simulink model "Quad_Linear_LQR"  (R2020a)
settings: Solver=ode4  StartTime=0.0  StopTime=10.0  FixedStep=0.01  RelTol=1e-3
InitFcn:
  | QuadConstants
undefined symbols (not defined in the file or in its folder): A1, A3, B1, B3, C2, Omega
settings Model: Creator=Ali  LastModifiedBy=Ali

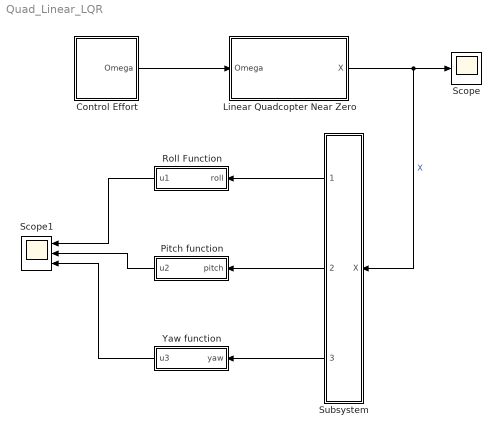
== system Quad_Linear_LQR ==
  Control Effort : Subsystem
  Linear Quadcopter Near Zero : Subsystem
  Pitch function : MATLAB Function  TreatAsAtomicUnit=on
  Roll Function : MATLAB Function  TreatAsAtomicUnit=on
  Scope : Scope
  Scope1 : Scope  NumInputPorts=3
  Subsystem : Subsystem
  Yaw function : MATLAB Function  TreatAsAtomicUnit=on
  wires:
  Control Effort/1(Omega) -> Linear Quadcopter Near Zero/1(Omega)
  Linear Quadcopter Near Zero/1(X) -> Subsystem/1(X), Scope/1  "X"
  Subsystem/1(roll) -> Roll Function/1(roll)
  Subsystem/2(pitch) -> Pitch function/1(pitch)
  Subsystem/3(yaw) -> Yaw function/1(yaw)
  Roll Function/1(u1) -> Scope1/1
  Pitch function/1(u2) -> Scope1/2
  Yaw function/1(u3) -> Scope1/3

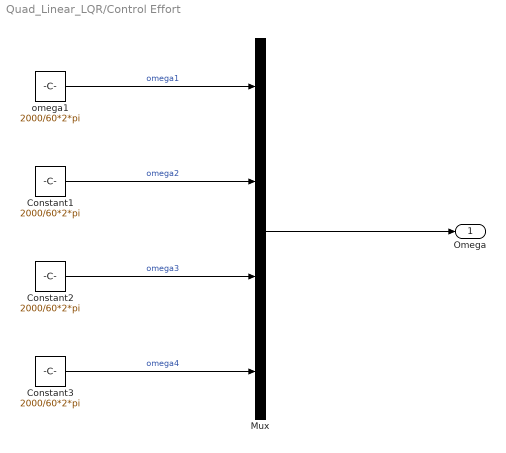
== system Quad_Linear_LQR/Control Effort ==
  Constant1 : Constant  Value=2000/60*2*pi
  Constant2 : Constant  Value=2000/60*2*pi
  Constant3 : Constant  Value=2000/60*2*pi
  Mux : Mux
  omega1 : Constant  Value=2000/60*2*pi
  Omega : Outport
  wires:
  Constant1/1 -> Mux/2  "omega2"
  Constant2/1 -> Mux/3  "omega3"
  Constant3/1 -> Mux/4  "omega4"
  omega1/1 -> Mux/1  "omega1"
  Mux/1 -> Omega/1

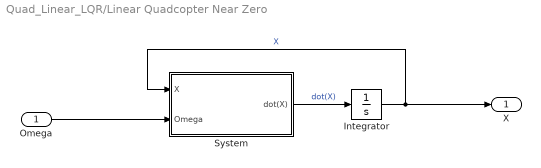
== system Quad_Linear_LQR/Linear Quadcopter Near Zero ==
  Omega : Inport
  Integrator : Integrator
  System : Subsystem
  X : Outport
  wires:
  Integrator/1 -> X/1, System/1(X)  "X"
  System/1(dot(X)) -> Integrator/1  "dot(X)"
  Omega/1 -> System/2(Omega)

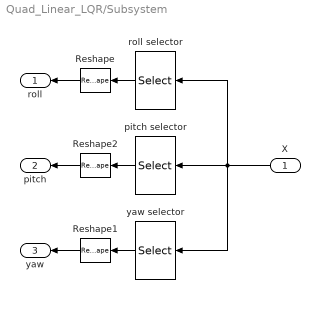
== system Quad_Linear_LQR/Subsystem ==
  X : Inport
  Reshape : Reshape  OutputDimensionality=Column vector (2-D)
  Reshape1 : Reshape  OutputDimensionality=Column vector (2-D)
  Reshape2 : Reshape  OutputDimensionality=Column vector (2-D)
  pitch selector : Selector  InputPortWidth=6  IndexOptions=Index vector (dialog)  Indices=[2 5]  OutputSizes=1
  roll selector : Selector  InputPortWidth=6  IndexOptions=Index vector (dialog)  Indices=[1 4]  OutputSizes=1
  yaw selector : Selector  InputPortWidth=6  IndexOptions=Index vector (dialog)  Indices=[3 6]  OutputSizes=1
  roll : Outport
  pitch : Outport  Port=2
  yaw : Outport  Port=3
  wires:
  X/1 -> yaw selector/1, roll selector/1, pitch selector/1
  roll selector/1 -> Reshape/1
  pitch selector/1 -> Reshape2/1
  yaw selector/1 -> Reshape1/1
  Reshape/1 -> roll/1
  Reshape2/1 -> pitch/1
  Reshape1/1 -> yaw/1

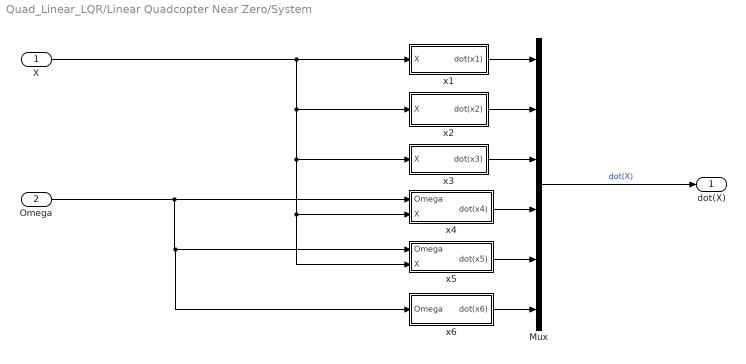
== system Quad_Linear_LQR/Linear Quadcopter Near Zero/System ==
  X : Inport
  Omega : Inport  Port=2
  Mux : Mux  Inputs=6
  x1 : Subsystem
  x2 : Subsystem
  x3 : Subsystem
  x4 : Subsystem
  x5 : Subsystem
  x6 : Subsystem
  dot(X) : Outport
  wires:
  Omega/1 -> x4/1(Omega), x6/1(Omega), x5/1(Omega)
  x6/1(dot(x6)) -> Mux/6
  x3/1(dot(x3)) -> Mux/3
  x4/1(dot(x4)) -> Mux/4
  x2/1(dot(x2)) -> Mux/2
  X/1 -> x5/2(X), x4/2(X), x3/1(X), x2/1(X), x1/1(X)
  x5/1(dot(x5)) -> Mux/5
  x1/1(dot(x1)) -> Mux/1
  Mux/1 -> dot(X)/1  "dot(X)"

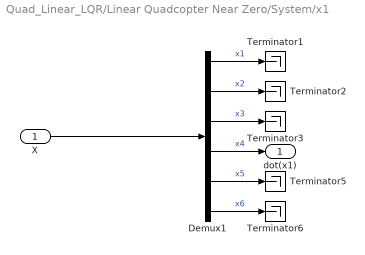
== system Quad_Linear_LQR/Linear Quadcopter Near Zero/System/x1 ==
  X : Inport
  Demux1 : Demux  Outputs=6
  Terminator{1..3,5..6} (5 alike) : Terminator
  dot(x1) : Outport
  wires:
  Demux1/4 -> dot(x1)/1  "x4"
  X/1 -> Demux1/1
  Demux1/6 -> Terminator6/1  "x6"
  Demux1/5 -> Terminator5/1  "x5"
  Demux1/3 -> Terminator3/1  "x3"
  Demux1/2 -> Terminator2/1  "x2"
  Demux1/1 -> Terminator1/1  "x1"

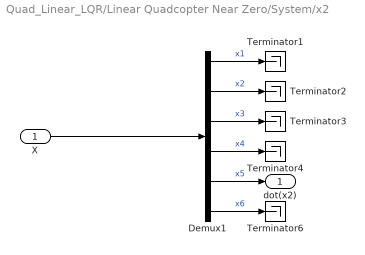
== system Quad_Linear_LQR/Linear Quadcopter Near Zero/System/x2 ==
  X : Inport
  Demux1 : Demux  Outputs=6
  Terminator{1..4,6} (5 alike) : Terminator
  dot(x2) : Outport
  wires:
  Demux1/4 -> Terminator4/1  "x4"
  X/1 -> Demux1/1
  Demux1/6 -> Terminator6/1  "x6"
  Demux1/5 -> dot(x2)/1  "x5"
  Demux1/3 -> Terminator3/1  "x3"
  Demux1/2 -> Terminator2/1  "x2"
  Demux1/1 -> Terminator1/1  "x1"

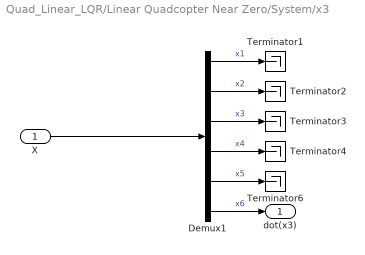
== system Quad_Linear_LQR/Linear Quadcopter Near Zero/System/x3 ==
  X : Inport
  Demux1 : Demux  Outputs=6
  Terminator{1..4,6} (5 alike) : Terminator
  dot(x3) : Outport
  wires:
  Demux1/4 -> Terminator4/1  "x4"
  X/1 -> Demux1/1
  Demux1/6 -> dot(x3)/1  "x6"
  Demux1/5 -> Terminator6/1  "x5"
  Demux1/3 -> Terminator3/1  "x3"
  Demux1/2 -> Terminator2/1  "x2"
  Demux1/1 -> Terminator1/1  "x1"

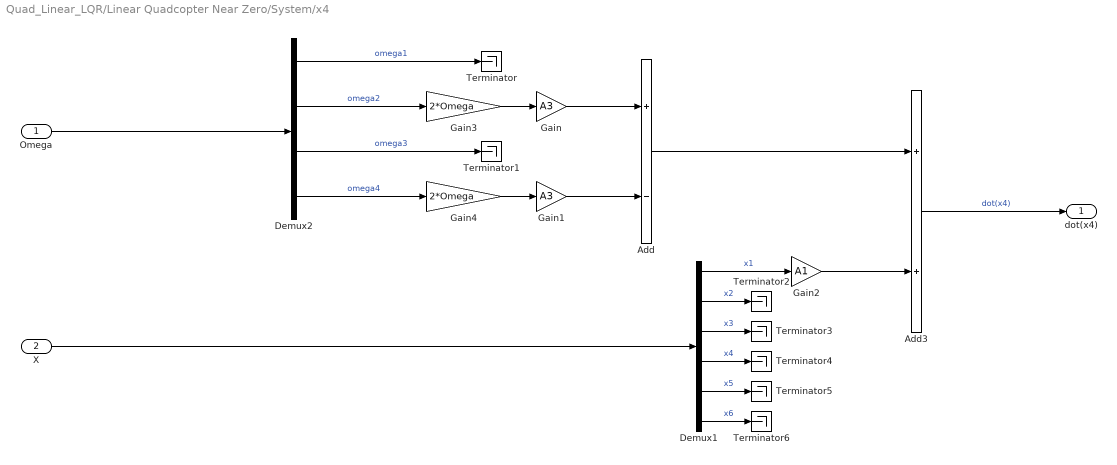
== system Quad_Linear_LQR/Linear Quadcopter Near Zero/System/x4 ==
  Omega : Inport
  X : Inport  Port=2
  Add : Sum  Inputs=+-
  Add3 : Sum
  Demux1 : Demux  Outputs=6
  Demux2 : Demux
  Gain : Gain  Gain=A3
  Gain1 : Gain  Gain=A3
  Gain2 : Gain  Gain=A1
  Gain3 : Gain  Gain=2*Omega
  Gain4 : Gain  Gain=2*Omega
  Terminator{,1..6} (7 alike) : Terminator
  dot(x4) : Outport
  wires:
  Gain2/1 -> Add3/2
  Gain1/1 -> Add/2
  Gain/1 -> Add/1
  Demux2/4 -> Gain4/1  "omega4"
  Demux2/2 -> Gain3/1  "omega2"
  Demux2/3 -> Terminator1/1  "omega3"
  Demux2/1 -> Terminator/1  "omega1"
  Demux1/5 -> Terminator5/1  "x5"
  Demux1/2 -> Terminator2/1  "x2"
  Demux1/3 -> Terminator3/1  "x3"
  Demux1/1 -> Gain2/1  "x1"
  Demux1/4 -> Terminator4/1  "x4"
  X/1 -> Demux1/1
  Demux1/6 -> Terminator6/1  "x6"
  Gain3/1 -> Gain/1
  Gain4/1 -> Gain1/1
  Omega/1 -> Demux2/1
  Add/1 -> Add3/1
  Add3/1 -> dot(x4)/1  "dot(x4)"

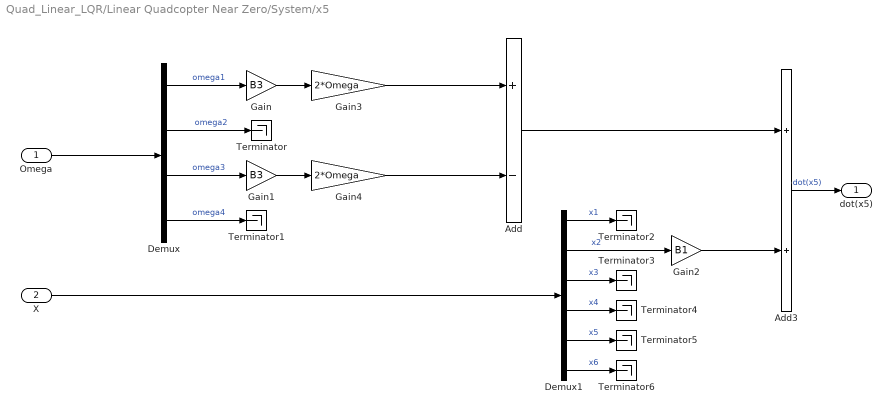
== system Quad_Linear_LQR/Linear Quadcopter Near Zero/System/x5 ==
  Omega : Inport
  X : Inport  Port=2
  Add : Sum  Inputs=+-
  Add3 : Sum
  Demux : Demux
  Demux1 : Demux  Outputs=6
  Gain : Gain  Gain=B3
  Gain1 : Gain  Gain=B3
  Gain2 : Gain  Gain=B1
  Gain3 : Gain  Gain=2*Omega
  Gain4 : Gain  Gain=2*Omega
  Terminator{,1..6} (7 alike) : Terminator
  dot(x5) : Outport
  wires:
  Gain1/1 -> Gain4/1
  Gain/1 -> Gain3/1
  Demux/2 -> Terminator/1  "omega2"
  Demux/4 -> Terminator1/1  "omega4"
  Demux/1 -> Gain/1  "omega1"
  Demux/3 -> Gain1/1  "omega3"
  Demux1/5 -> Terminator5/1  "x5"
  Demux1/2 -> Gain2/1  "x2"
  Demux1/3 -> Terminator3/1  "x3"
  Demux1/1 -> Terminator2/1  "x1"
  Demux1/4 -> Terminator4/1  "x4"
  X/1 -> Demux1/1
  Demux1/6 -> Terminator6/1  "x6"
  Gain3/1 -> Add/1
  Gain4/1 -> Add/2
  Omega/1 -> Demux/1
  Add/1 -> Add3/1
  Gain2/1 -> Add3/2
  Add3/1 -> dot(x5)/1  "dot(x5)"

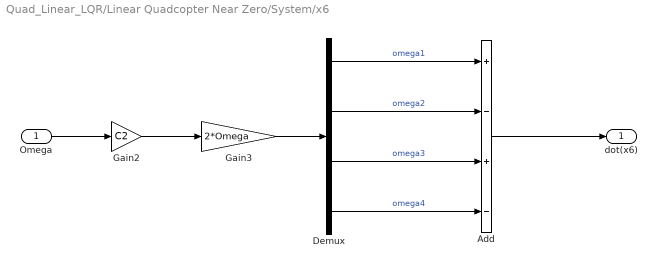
== system Quad_Linear_LQR/Linear Quadcopter Near Zero/System/x6 ==
  Omega : Inport
  Add : Sum  Inputs=+-+-
  Demux : Demux
  Gain2 : Gain  Gain=C2
  Gain3 : Gain  Gain=2*Omega
  dot(x6) : Outport
  wires:
  Omega/1 -> Gain2/1
  Demux/1 -> Add/1  "omega1"
  Demux/2 -> Add/2  "omega2"
  Demux/3 -> Add/3  "omega3"
  Demux/4 -> Add/4  "omega4"
  Add/1 -> dot(x6)/1
  Gain3/1 -> Demux/1
  Gain2/1 -> Gain3/1

== matlab function Quad_Linear_LQR/Roll Function ==
  data: roll input; u1 output
function u1 = fcn(roll)
% QuadConstants;
%%% constans %%%
% Distance between rotor center to quad center (m)
d_cg = 0.295;
% Distance between D point to quad center (m)
h_cg = 0.0078;
% Thrust factor (non dimensional)
b = 1.10794e-5;
% Rotor torque drag factor (non dimensional)
d = 3.2e-6;
% Total mass (kg)
m_tot = 1.774;
% Quad Moment of inertia respect to axix X Body (kg.m^2)
J_xx = 0.0297598;
% Quad Moment of inertia respect to axix Y Body (kg.m^2)
J_yy = 0.0298565;
% Quad Moment of inertia respect to axix Y Body (kg.m^2)
J_zz = 0.058510;
% Quad blade Moment (kg.m^2)
J_R = 4.439e-5;
% Mass on X axis bearing (kg)
m1 = 1.272;
% Mass on Y axis bearing (kg)
m2 = 1.074;
% Mass on Z axis bearing (kg)
m3 = 1.693;
% Bearing radius in X axix (m)
r_x = 0.01;
% Bearing radius in Y axix (m)
r_y = 0.01;
% Bearing radius in Z axix (m)
r_z = 0.025;
% Static bearing friction (non dimensional)
% miu_s = 0.003;
% Dynamic bearing friction (non dimensional)
miu_k = 0.002;
% Motor constant (non dimensional)
% tau = 0.15;
% Delay of motor (sec)
% T_d = 0.02;
% Gravity force (m/s^2)
g = 9.81;
% A Constants
A1 = (h_cg * g * m_tot) / (m_tot * h_cg^2 + J_xx);
A2 = (2*m_tot * h_cg^2 + J_yy -J_zz) / (m_tot * h_cg^2 + J_xx);
A3 = (b * d_cg) / (m_tot * h_cg^2 + J_xx);
A4 = (J_R) / (m_tot * h_cg^2 + J_xx);
A5 = (m1 * g * miu_k * r_x) / (m_tot * h_cg^2 + J_xx);
% B Constants
B1 = (h_cg * g * m_tot) / (m_tot * h_cg^2 + J_yy);
B2 = (-2*m_tot * h_cg^2 - J_xx + J_zz) / (m_tot * h_cg^2 + J_yy);
B3 = (b * d_cg) / (m_tot * h_cg^2 + J_yy);
B4 = (-J_R) / (m_tot * h_cg^2 + J_yy);
B5 = (m2 * g * miu_k * r_y) / (m_tot * h_cg^2 + J_yy);
% C Constants
C1 = (J_xx - J_yy) / (J_zz);
C2 = (d) / (J_zz);
C3 = (m3 * g * miu_k * r_z) / (J_zz);
% omega for linearzation 2000 RPM
Omega = 2000 / 60 * 2 * pi;

x1     = roll(1);
A11    = 0; %da1dx1
A14    = 1; %da1dx4
A41    = A1 * cos(x1); %da4dx1
A44    = 0; %da4dx4

A      = [A11, A14 ;
          A41, A44];
B      = [0  ;
          A3];
a      = A(2);
b      = B(2);

q1     = 10;
q2     = 10;
R      = 1;
R_inv  = R^-1;
K_ans = zeros(2, 2);
% algebraic_riccati = K * A + A' * K - K * B * R^-1 * B' * K + Q;
% first equation q1 + 2*a*k12 - (b^2*k12^2)/R = 0
% Ans1 K12 = -m*(k + (k^2 + Q11)^(1/2))
% Ans2 K12 = -m*(k - (k^2 + Q11)^(1/2))
K12 = zeros(1, 2);
K12(1) = (R*(a + ((R*a^2 + q1*b^2)/R)^(1/2)))/b^2;
K12(2) = (R*(a - ((R*a^2 + q1*b^2)/R)^(1/2)))/b^2;
for i = 1:length(K12)
    if ~isreal(K12(i))
        continue;
    end
    % Second equation 2*k12 + q2 - (b^2*k22^2)/R = 0
    % Ans1 K12 =  (2*k12 + q2)^(1/2)/(R^(1/2)*b)
    % Ans2 K12 = -(2*k12 + q2)^(1/2)/(R^(1/2)*b)
    K22 = zeros(1, 2);
    K22(1) =  (R^(1/2)*(2*K12(i) + q2)^(1/2))/b;
    K22(2) = -(R^(1/2)*(2*K12(i) + q2)^(1/2))/b;
    for j = 1:length(K22)
        if ~isreal(K22(j))
            continue
        end
        % Last equation k11 + a*k22 - (b^2*k12*k22)/R = 0
        % Ans R*k12*k22*b^2 - a*k22
        K11 = (K12(i)*K22(j)*b^2)/R - a*K22(j);
        temp_K = zeros(2, 2);
        temp_K(1, 1) = K11;
        temp_K(1, 2) = K12(i);
        temp_K(2, 1) = K12(i);
        temp_K(2, 2) = K22(j);
        if all(eig(A - B * R^(-1)* B' * temp_K) < 0)
            K_ans = temp_K;
            break;
        end
    end
end

u1 = -R_inv*B'*K_ans*roll;

== matlab function Quad_Linear_LQR/Yaw function ==
  data: yaw input; u3 output
function u3 = fcn(yaw)
% QuadConstants;
%%% constans %%%
% Distance between rotor center to quad center (m)
d_cg = 0.295;
% Distance between D point to quad center (m)
h_cg = 0.0078;
% Thrust factor (non dimensional)
b = 1.10794e-5;
% Rotor torque drag factor (non dimensional)
d = 3.2e-6;
% Total mass (kg)
m_tot = 1.774;
% Quad Moment of inertia respect to axix X Body (kg.m^2)
J_xx = 0.0297598;
% Quad Moment of inertia respect to axix Y Body (kg.m^2)
J_yy = 0.0298565;
% Quad Moment of inertia respect to axix Y Body (kg.m^2)
J_zz = 0.058510;
% Quad blade Moment (kg.m^2)
J_R = 4.439e-5;
% Mass on X axis bearing (kg)
m1 = 1.272;
% Mass on Y axis bearing (kg)
m2 = 1.074;
% Mass on Z axis bearing (kg)
m3 = 1.693;
% Bearing radius in X axix (m)
r_x = 0.01;
% Bearing radius in Y axix (m)
r_y = 0.01;
% Bearing radius in Z axix (m)
r_z = 0.025;
% Static bearing friction (non dimensional)
% miu_s = 0.003;
% Dynamic bearing friction (non dimensional)
miu_k = 0.002;
% Motor constant (non dimensional)
% tau = 0.15;
% Delay of motor (sec)
% T_d = 0.02;
% Gravity force (m/s^2)
g = 9.81;
% A Constants
A1 = (h_cg * g * m_tot) / (m_tot * h_cg^2 + J_xx);
A2 = (2*m_tot * h_cg^2 + J_yy -J_zz) / (m_tot * h_cg^2 + J_xx);
A3 = (b * d_cg) / (m_tot * h_cg^2 + J_xx);
A4 = (J_R) / (m_tot * h_cg^2 + J_xx);
A5 = (m1 * g * miu_k * r_x) / (m_tot * h_cg^2 + J_xx);
% B Constants
B1 = (h_cg * g * m_tot) / (m_tot * h_cg^2 + J_yy);
B2 = (-2*m_tot * h_cg^2 - J_xx + J_zz) / (m_tot * h_cg^2 + J_yy);
B3 = (b * d_cg) / (m_tot * h_cg^2 + J_yy);
B4 = (-J_R) / (m_tot * h_cg^2 + J_yy);
B5 = (m2 * g * miu_k * r_y) / (m_tot * h_cg^2 + J_yy);
% C Constants
C1 = (J_xx - J_yy) / (J_zz);
C2 = (d) / (J_zz);
C3 = (m3 * g * miu_k * r_z) / (J_zz);
% omega for linearzation 2000 RPM
Omega = 2000 / 60 * 2 * pi;

A33    = 0; %da3dx3
A36    = 1; %da3dx6
A63    = 0; %da6dx3
A66    = 0; %da6dx6


A      = [A33, A36 ;
          A63, A66];
B      = [0  ;
          C2];
a      = A(2);
b      = B(2);

q1     = 100000;
q2     = 100000;
R      = 1;
R_inv  = R^-1;
K_ans = zeros(2, 2);
% algebraic_riccati = K * A + A' * K - K * B * R^-1 * B' * K + Q;
% first equation q1 + 2*a*k12 - (b^2*k12^2)/R = 0
% Ans1 K12 = -m*(k + (k^2 + Q11)^(1/2))
% Ans2 K12 = -m*(k - (k^2 + Q11)^(1/2))
K12 = zeros(1, 2);
K12(1) = (R*(a + ((R*a^2 + q1*b^2)/R)^(1/2)))/b^2;
K12(2) = (R*(a - ((R*a^2 + q1*b^2)/R)^(1/2)))/b^2;
for i = 1:length(K12)
    if ~isreal(K12(i))
        continue;
    end
    % Second equation 2*k12 + q2 - (b^2*k22^2)/R = 0
    % Ans1 K12 =  (2*k12 + q2)^(1/2)/(R^(1/2)*b)
    % Ans2 K12 = -(2*k12 + q2)^(1/2)/(R^(1/2)*b)
    K22 = zeros(1, 2);
    if 2*K12(i) + q2 >= 0
        K22(1) =  (R^(1/2)*(2*K12(i) + q2)^(1/2))/b;
    else
        K22(1) =  complex(0, 1);
    end
    K22(2) = -(R^(1/2)*(2*K12(i) + q2)^(1/2))/b;
    for j = 1:length(K22)
        if ~isreal(K22(j))
            continue
        end
        % Last equation k11 + a*k22 - (b^2*k12*k22)/R = 0
        % Ans R*k12*k22*b^2 - a*k22
        K11 = (K12(i)*K22(j)*b^2)/R - a*K22(j);
        temp_K = zeros(2, 2);
        temp_K(1, 1) = K11;
        temp_K(1, 2) = K12(i);
        temp_K(2, 1) = K12(i);
        temp_K(2, 2) = K22(j);
        if all(eig(A - B * R^(-1)* B' * temp_K) < 0)
            K_ans = temp_K;
            break;
        end
    end
end

u3 = -R_inv*B'*K_ans*yaw;

== matlab function Quad_Linear_LQR/Pitch function ==
  data: pitch input; u2 output
function u2 = fcn(pitch)
% QuadConstants;
% QuadConstants;
%%% constans %%%
% Distance between rotor center to quad center (m)
d_cg = 0.295;
% Distance between D point to quad center (m)
h_cg = 0.0078;
% Thrust factor (non dimensional)
b = 1.10794e-5;
% Rotor torque drag factor (non dimensional)
d = 3.2e-6;
% Total mass (kg)
m_tot = 1.774;
% Quad Moment of inertia respect to axix X Body (kg.m^2)
J_xx = 0.0297598;
% Quad Moment of inertia respect to axix Y Body (kg.m^2)
J_yy = 0.0298565;
% Quad Moment of inertia respect to axix Y Body (kg.m^2)
J_zz = 0.058510;
% Quad blade Moment (kg.m^2)
J_R = 4.439e-5;
% Mass on X axis bearing (kg)
m1 = 1.272;
% Mass on Y axis bearing (kg)
m2 = 1.074;
% Mass on Z axis bearing (kg)
m3 = 1.693;
% Bearing radius in X axix (m)
r_x = 0.01;
% Bearing radius in Y axix (m)
r_y = 0.01;
% Bearing radius in Z axix (m)
r_z = 0.025;
% Static bearing friction (non dimensional)
% miu_s = 0.003;
% Dynamic bearing friction (non dimensional)
miu_k = 0.002;
% Motor constant (non dimensional)
% tau = 0.15;
% Delay of motor (sec)
% T_d = 0.02;
% Gravity force (m/s^2)
g = 9.81;
% A Constants
A1 = (h_cg * g * m_tot) / (m_tot * h_cg^2 + J_xx);
A2 = (2*m_tot * h_cg^2 + J_yy -J_zz) / (m_tot * h_cg^2 + J_xx);
A3 = (b * d_cg) / (m_tot * h_cg^2 + J_xx);
A4 = (J_R) / (m_tot * h_cg^2 + J_xx);
A5 = (m1 * g * miu_k * r_x) / (m_tot * h_cg^2 + J_xx);
% B Constants
B1 = (h_cg * g * m_tot) / (m_tot * h_cg^2 + J_yy);
B2 = (-2*m_tot * h_cg^2 - J_xx + J_zz) / (m_tot * h_cg^2 + J_yy);
B3 = (b * d_cg) / (m_tot * h_cg^2 + J_yy);
B4 = (-J_R) / (m_tot * h_cg^2 + J_yy);
B5 = (m2 * g * miu_k * r_y) / (m_tot * h_cg^2 + J_yy);
% C Constants
C1 = (J_xx - J_yy) / (J_zz);
C2 = (d) / (J_zz);
C3 = (m3 * g * miu_k * r_z) / (J_zz);
% omega for linearzation 2000 RPM
Omega = 2000 / 60 * 2 * pi;

x2     = pitch(1);
A22    = 0; %da2dx2
A25    = 1; %da2dx5
A52    = B1 * cos(x2); %da5dx2
A55    = 0; %da5dx5

A      = [A22, A25 ;
          A52, A55];
B      = [0  ;
          B3];
a      = A(2);
b      = B(2);

q1     = 10;
q2     = 10;
R      = 1;
R_inv  = R^-1;
K_ans = zeros(2, 2);
% algebraic_riccati = K * A + A' * K - K * B * R^-1 * B' * K + Q;
% first equation q1 + 2*a*k12 - (b^2*k12^2)/R = 0
% Ans1 K12 = -m*(k + (k^2 + Q11)^(1/2))
% Ans2 K12 = -m*(k - (k^2 + Q11)^(1/2))
K12 = zeros(1, 2);
K12(1) = (R*(a + ((R*a^2 + q1*b^2)/R)^(1/2)))/b^2;
K12(2) = (R*(a - ((R*a^2 + q1*b^2)/R)^(1/2)))/b^2;
for i = 1:length(K12)
    if ~isreal(K12(i))
        continue;
    end
    % Second equation 2*k12 + q2 - (b^2*k22^2)/R = 0
    % Ans1 K12 =  (2*k12 + q2)^(1/2)/(R^(1/2)*b)
    % Ans2 K12 = -(2*k12 + q2)^(1/2)/(R^(1/2)*b)
    K22 = zeros(1, 2);
    K22(1) =  (R^(1/2)*(2*K12(i) + q2)^(1/2))/b;
    K22(2) = -(R^(1/2)*(2*K12(i) + q2)^(1/2))/b;
    for j = 1:length(K22)
        if ~isreal(K22(j))
            continue
        end
        % Last equation k11 + a*k22 - (b^2*k12*k22)/R = 0
        % Ans R*k12*k22*b^2 - a*k22
        K11 = (K12(i)*K22(j)*b^2)/R - a*K22(j);
        temp_K = zeros(2, 2);
        temp_K(1, 1) = K11;
        temp_K(1, 2) = K12(i);
        temp_K(2, 1) = K12(i);
        temp_K(2, 2) = K22(j);
        if all(eig(A - B * R^(-1)* B' * temp_K) < 0)
            K_ans = temp_K;
            break;
        end
    end
end

u2 = -R_inv*B'*K_ans*pitch;
